simulink model "final_invpend_KunalJain_R2015a"  (R2015a)
settings: Solver=ode4  StartTime=0.0  StopTime=50  FixedStep=1e-4  RelTol=1e-5
libraries: simulink x2
settings Model: Creator=Aranya Dan  LastModifiedBy=Kunal
settings SolverCC: AlgebraicLoopSolver=LineSearch
settings DebuggingCC: MaxConsecutiveZCsMsg=none

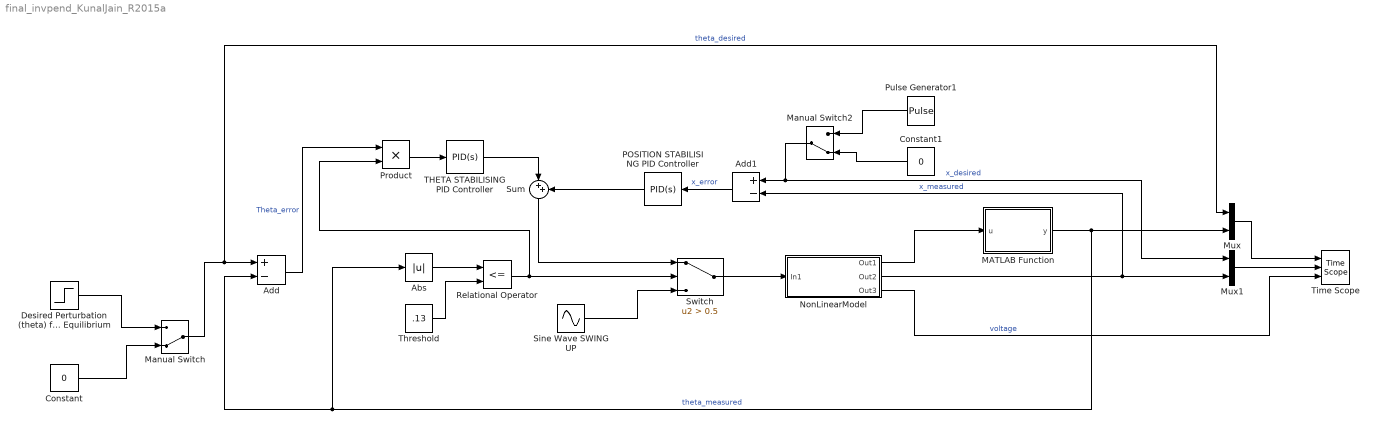
== system final_invpend_KunalJain_R2015a ==
  Abs : Abs
  Add : Sum  Inputs=+-
  Add1 : Sum  Inputs=+-
  Constant : Constant  Value=0
  Constant1 : Constant  Value=0
  Desired Perturbation (theta) from Equilibrium : Step  Time=40  After=0.12  SampleTime=0
  MATLAB Function : MATLAB Function  TreatAsAtomicUnit=on
  Manual Switch : ManualSwitch  CurrentSetting=0
  Manual Switch2 : ManualSwitch  CurrentSetting=0
  Mux : Mux  Inputs=2
  Mux1 : Mux  Inputs=2
  "NonLinearModel " : Subsystem
  POSITION STABILISING PID Controller : simulink/Continuous/PID Controller  Controller=PID  TimeDomain=Continuous-time  SampleTime=-1  IntegratorMethod=Forward Euler  FilterMethod=Forward Euler  Form=Parallel  UseFilter=on  ControllerParametersSource=internal  P=150  I=35  D=-95  N=1.6  InitialConditionSource=internal  InitialConditionForIntegrator=0  InitialConditionForFilter=0  ExternalReset=none  LimitOutput=off  UpperSaturationLimit=inf  LowerSaturationLimit=-inf  LinearizeAsGain=on  AntiWindupMode=none  Kb=1  TrackingMode=off  Kt=1  PParamMin=[]  PParamMax=[]  IParamMin=[]  IParamMax=[]  DParamMin=[]  DParamMax=[]  NParamMin=[]  NParamMax=[]  KbParamMin=[]  KbParamMax=[]  KtParamMin=[]  KtParamMax=[]  POutMin=[]  POutMax=[]  IOutMin=[]  IOutMax=[]  DOutMin=[]  DOutMax=[]  NOutMin=[]  NOutMax=[]  KbOutMin=[]  KbOutMax=[]  KtOutMin=[]  KtOutMax=[]  IntegratorOutMin=[]  IntegratorOutMax=[]  FilterOutMin=[]  FilterOutMax=[]  SumOutMin=[]  SumOutMax=[]  SumI1OutMin=[]  SumI1OutMax=[]  SumI2OutMin=[]  SumI2OutMax=[]  SumI3OutMin=[]  SumI3OutMax=[]  SumDOutMin=[]  SumDOutMax=[]  SaturationOutMin=[]  SaturationOutMax=[]  IntegratorContinuousStateAttributes=''  IntegratorStateMustResolveToSignalObject=off  IntegratorRTWStateStorageClass=Auto  FilterContinuousStateAttributes=''  FilterStateMustResolveToSignalObject=off  FilterRTWStateStorageClass=Auto  DifferentiatorICPrevScaledInput=0  DifferentiatorOutMin=[]  DifferentiatorOutMax=[]
  Product : Product
  Pulse Generator1 : DiscretePulseGenerator  PulseType=Time based  Amplitude=0.1
  Relational Operator : RelationalOperator  Operator=<=  OutDataTypeStr=boolean
  Sine Wave SWING UP : Sin  Amplitude=1.75  Frequency=2.1011  Phase=pi/2  SampleTime=0
  Sum : Sum  Inputs=|++
  Switch : Switch  Criteria=u2 > Threshold  Threshold=0.5
  THETA STABILISING PID Controller : simulink/Continuous/PID Controller  Controller=PID  TimeDomain=Continuous-time  SampleTime=-1  IntegratorMethod=Forward Euler  FilterMethod=Forward Euler  Form=Parallel  UseFilter=on  ControllerParametersSource=internal  P=225  I=5926  D=2.123  N=8346  InitialConditionSource=internal  InitialConditionForIntegrator=0  InitialConditionForFilter=0  ExternalReset=none  LimitOutput=off  UpperSaturationLimit=inf  LowerSaturationLimit=-inf  LinearizeAsGain=on  AntiWindupMode=none  Kb=1  TrackingMode=off  Kt=1  PParamMin=[]  PParamMax=[]  IParamMin=[]  IParamMax=[]  DParamMin=[]  DParamMax=[]  NParamMin=[]  NParamMax=[]  KbParamMin=[]  KbParamMax=[]  KtParamMin=[]  KtParamMax=[]  POutMin=[]  POutMax=[]  IOutMin=[]  IOutMax=[]  DOutMin=[]  DOutMax=[]  NOutMin=[]  NOutMax=[]  KbOutMin=[]  KbOutMax=[]  KtOutMin=[]  KtOutMax=[]  IntegratorOutMin=[]  IntegratorOutMax=[]  FilterOutMin=[]  FilterOutMax=[]  SumOutMin=[]  SumOutMax=[]  SumI1OutMin=[]  SumI1OutMax=[]  SumI2OutMin=[]  SumI2OutMax=[]  SumI3OutMin=[]  SumI3OutMax=[]  SumDOutMin=[]  SumDOutMax=[]  SaturationOutMin=[]  SaturationOutMax=[]  IntegratorContinuousStateAttributes=''  IntegratorStateMustResolveToSignalObject=off  IntegratorRTWStateStorageClass=Auto  FilterContinuousStateAttributes=''  FilterStateMustResolveToSignalObject=off  FilterRTWStateStorageClass=Auto  DifferentiatorICPrevScaledInput=0  DifferentiatorOutMin=[]  DifferentiatorOutMax=[]
  Threshold : Constant  Value=.13
  Time Scope : TimeScope  DefaultConfigurationName=spbscopes.TimeScopeBlockCfg  NumInputPorts=3
  wires:
  "NonLinearModel "/1(Out1) -> MATLAB Function/1(u)
  Mux/1 -> Time Scope/1
  Abs/1 -> Relational Operator/1
  Threshold/1 -> Relational Operator/2
  Relational Operator/1 -> Switch/2, Product/2
  "NonLinearModel "/2(Out2) -> Mux1/2, Add1/2  "x_measured"
  Add/1 -> Product/1  "Theta_error"
  "NonLinearModel "/3(Out3) -> Time Scope/3  "voltage"
  Constant/1 -> Manual Switch/2
  Desired Perturbation (theta) from Equilibrium/1 -> Manual Switch/1
  Manual Switch/1 -> Add/1, Mux/1  "theta_desired"
  MATLAB Function/1(y) -> Add/2, Abs/1, Mux/2  "theta_measured"
  Switch/1 -> "NonLinearModel "/1(In1)
  Add1/1 -> POSITION STABILISING PID Controller/1  "x_error"
  Pulse Generator1/1 -> Manual Switch2/1
  Manual Switch2/1 -> Mux1/1, Add1/1  "x_desired"
  Constant1/1 -> Manual Switch2/2
  THETA STABILISING PID Controller/1 -> Sum/1
  Sum/1 -> Switch/1
  Sine Wave SWING UP/1 -> Switch/3
  Product/1 -> THETA STABILISING PID Controller/1
  POSITION STABILISING PID Controller/1 -> Sum/2
  Mux1/1 -> Time Scope/2

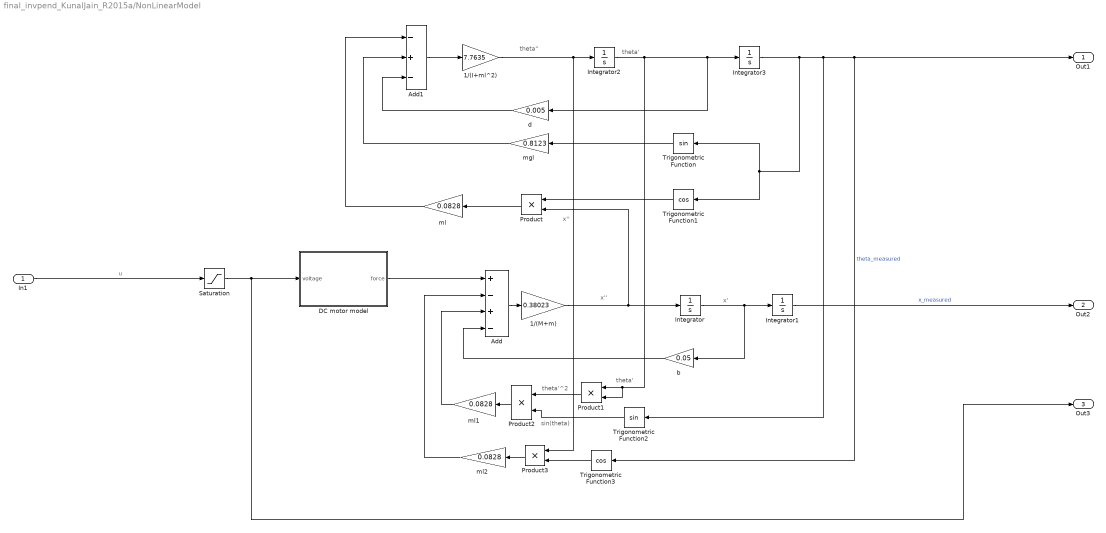
== system final_invpend_KunalJain_R2015a/NonLinearModel  ==
  note: theta''
  note: x''
  note: theta'
  note: x'
  note: x''
  note: theta'
  note: sin(theta)
  note: theta'^2
  In1 : Inport
  1/(I+ml^2) : Gain  Gain=7.7635
  1/(M+m) : Gain  Gain=0.38023
  Add : Sum  Inputs=+-+-
  Add1 : Sum  Inputs=-+-
  DC motor model : Subsystem
  Integrator : Integrator
  Integrator1 : Integrator
  Integrator2 : Integrator
  Integrator3 : Integrator  InitialCondition=pi
  Product{,1..3} (4 alike) : Product
  Saturation : Saturate  UpperLimit=6  LowerLimit=-6
  Trigonometric Function : Trigonometry
  Trigonometric Function1 : Trigonometry  Operator=cos
  Trigonometric Function2 : Trigonometry
  Trigonometric Function3 : Trigonometry  Operator=cos
  b : Gain  Gain=0.05
  d : Gain  Gain=0.005
  mgl : Gain  Gain=0.8123
  ml : Gain  Gain=0.0828
  ml1 : Gain  Gain=0.0828
  ml2 : Gain  Gain=0.0828
  Out1 : Outport
  Out2 : Outport  Port=2
  Out3 : Outport  Port=3
  wires:
  In1/1 -> Saturation/1  "u"
  1/(M+m)/1 -> Product/2, Integrator/1
  Add1/1 -> 1/(I+ml^2)/1
  Integrator3/1 -> Trigonometric Function2/1, Trigonometric Function3/1, Out1/1, Trigonometric Function1/1, Trigonometric Function/1  "theta_measured"
  Integrator/1 -> b/1, Integrator1/1
  Integrator1/1 -> Out2/1  "x_measured"
  b/1 -> Add/4
  mgl/1 -> Add1/2
  Add/1 -> 1/(M+m)/1
  ml2/1 -> Add/2
  ml1/1 -> Add/3
  Trigonometric Function/1 -> mgl/1
  ml/1 -> Add1/1
  Product/1 -> ml/1
  Trigonometric Function1/1 -> Product/1
  d/1 -> Add1/3
  DC motor model/1(force) -> Add/1
  Integrator2/1 -> Product1/2, Product1/1, d/1, Integrator3/1
  Product1/1 -> Product2/1
  Product2/1 -> ml1/1
  Trigonometric Function2/1 -> Product2/2
  Product3/1 -> ml2/1
  1/(I+ml^2)/1 -> Integrator2/1, Product3/1
  Trigonometric Function3/1 -> Product3/2
  Saturation/1 -> Out3/1, DC motor model/1(voltage)

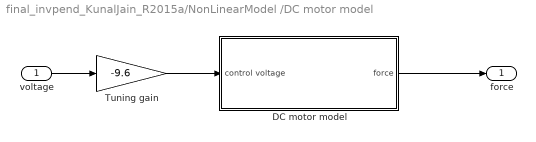
== system final_invpend_KunalJain_R2015a/NonLinearModel /DC motor model ==
  voltage : Inport
  DC motor model : Subsystem  mask{J=0.0000140, Kt=0.05, Kb=0.05, d=0.000001, R=2.5, L=0.0025}
      mask prompts: J "Moment of inertia"; Kt "Torque constant"; Kb "Electromotive force constant"; d "Linear approximation of viscous friction"; R "Electrical circuit resistance"; L "Electrical circuit inductance"
      mask Display: disp('DC motor')
  Tuning gain : Gain  Gain=-9.6
  force : Outport
  wires:
  DC motor model/1(force) -> force/1
  voltage/1 -> Tuning gain/1
  Tuning gain/1 -> DC motor model/1(control voltage)

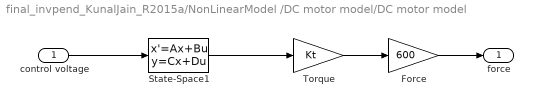
== system final_invpend_KunalJain_R2015a/NonLinearModel /DC motor model/DC motor model ==
  control voltage : Inport
  Force : Gain  Gain=600
  State-Space1 : StateSpace  A=[-d/J Kt/J;-Kb/L -R/L]  B=[0; 1/L]  C=[0 1]  D=0  X0=0
  Torque : Gain  Gain=Kt
  force : Outport
  wires:
  Force/1 -> force/1
  Torque/1 -> Force/1
  State-Space1/1 -> Torque/1
  control voltage/1 -> State-Space1/1

== matlab function final_invpend_KunalJain_R2015a/MATLAB Function ==
  data: u input; y output
function y = fcn(u)
%#codegen
y=mod(u+pi,2*pi)-pi;
end
